simulink model "peloel"  (R2023b)
settings: Solver=VariableStepAuto  StartTime=0.0  StopTime=0.1  RelTol=1e-3
libraries: spsMosfetLib x4, spsDCVoltageSourceLib x1, spsSeriesRLCBranchLib x1, spsVoltageMeasurementLib x1, sps_lib x1
settings Model: Creator=ayesh  LastModifiedBy=ayesh

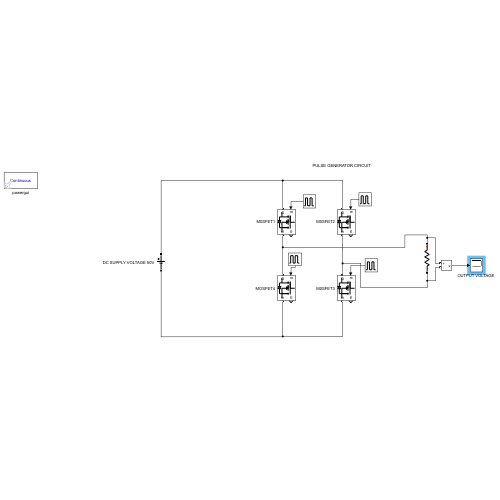
[thumbnail: Simulink's stored preview of the top-level diagram]
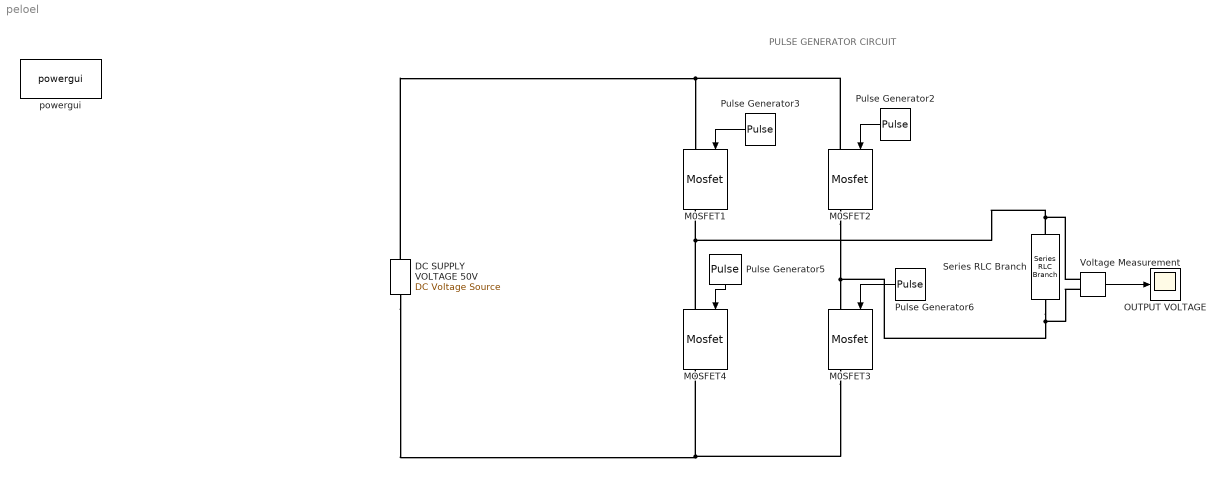
== system peloel ==
  note: PULSE GENERATOR CIRCUIT
  DC SUPPLY VOLTAGE 50V : spsDCVoltageSourceLib/DC Voltage Source  Amplitude=5  Measurements=None
  M0SFET1 : spsMosfetLib/Mosfet  Ron=0.1  Lon=0  Rd=0.01  Vfd=0  IC=0  Rs=1e5  Cs=inf  Measurements=on
  M0SFET2 : spsMosfetLib/Mosfet  Ron=0.1  Lon=0  Rd=0.01  Vfd=0  IC=0  Rs=1e5  Cs=inf  Measurements=on
  M0SFET3 : spsMosfetLib/Mosfet  Ron=0.1  Lon=0  Rd=0.01  Vfd=0  IC=0  Rs=1e5  Cs=inf  Measurements=on
  MOSFET4 : spsMosfetLib/Mosfet  Ron=0.1  Lon=0  Rd=0.01  Vfd=0  IC=0  Rs=1e5  Cs=inf  Measurements=on
  "OUTPUT VOLTAGE " : Scope
  Pulse Generator2 : DiscretePulseGenerator  PulseType=Time based  Period=0.016666666  PulseWidth=50  PhaseDelay=0.00555555555
  Pulse Generator3 : DiscretePulseGenerator  PulseType=Time based  Period=0.01666666  PulseWidth=50
  Pulse Generator5 : DiscretePulseGenerator  PulseType=Time based  Period=0.01666666  PulseWidth=50  PhaseDelay=0.0083333
  Pulse Generator6 : DiscretePulseGenerator  PulseType=Time based  Period=0.0166666666  PulseWidth=50  PhaseDelay=0.01388888888
  Series RLC Branch : spsSeriesRLCBranchLib/Series RLC Branch  LConnTagsString=__new0  RConnTagsString=__new0  BranchType=R  Resistance=50  Inductance=1e-3  SetiL0=off  InitialCurrent=0  Capacitance=1e-6  Setx0=off  InitialVoltage=0  Measurements=None
  Voltage Measurement : spsVoltageMeasurementLib/Voltage Measurement  PhasorSimulation=off  OutputType=Complex  PSBequivalent=0
  powergui : sps_lib/powergui  Priority=1  SimulationMode=Continuous  SampleTime=50e-6  frequency=60  Iterations=50  frequencyindice=0  Pbase=100e6  ErrMax=1e-4  UnitsV=kV  UnitsW=MW  buscounter=0  FunctionMessages=off  echomessages=off  EnableUseOfTLC=off  CurrentSourceSwitches=off  DisableSnubberDevices=off  DisableRonSwitches=off  DisableVfSwitches=off  DisplayEquations=off  AutomaticDiscreteSolvers=off  SolverType=Tustin/Backward Euler (TBE)  Interpol=off  ExternalGateDelay=off  methode=off  Ts=100  x0status=blocks  SPID=on  SwTol=0  HookPort=off  NonlinearTolerance=1e-4  nMaxIteration=100  ContinueOnMaxIteration=off  RestoreLinks=warning  ResistiveCurrentMeasurement=off  Frange=[0:2:500]  Ylog=off  Xlog=on  ShowGrid=off  save=off  variable=ZData  structure=0  ZoomFFT=off  StartTime=0.0  cycles=1  DisplayStyle=1  fundamental=60  FreqAxis=off  MaxFrequency=1000  frequencyindicesteady=1  RmsSteady=1  display=off
  wires:
  Voltage Measurement/1 -> "OUTPUT VOLTAGE "/1
  Pulse Generator6/1 -> M0SFET3/1
  Pulse Generator2/1 -> M0SFET2/1
  Pulse Generator3/1 -> M0SFET1/1
  Pulse Generator5/1 -> MOSFET4/1
  connections:
  DC SUPPLY VOLTAGE 50V/RConn1 -- M0SFET2/LConn1 -- M0SFET1/LConn1
  MOSFET4/LConn1 -- Voltage Measurement/LConn1 -- Series RLC Branch/LConn1 -- M0SFET1/RConn1
  DC SUPPLY VOLTAGE 50V/LConn1 -- M0SFET3/RConn1 -- MOSFET4/RConn1
  M0SFET2/RConn1 -- Voltage Measurement/LConn2 -- Series RLC Branch/RConn1 -- M0SFET3/LConn1
